simulink model "TCU_Final"  (R2025b)
settings: Solver=FixedStepDiscrete  StartTime=0.0  StopTime=inf  RelTol=1e-3
libraries: TCU_GS x1, TCU_HPC x1
settings Model: Creator=Jairs  LastModifiedBy=joshu
settings OptimizationCC: DefaultParameterBehavior=Inlined  EnhancedBackFolding=on  PassReuseOutputArgsAs=Individual arguments  ZeroExternalMemoryAtStartup=off  ZeroInternalMemoryAtStartup=off  OptimizeBlockOrder=speed  DifferentSizesBufferReuse=on  OptimizationCustomize=off  EfficientTunableParamExpr=on
settings DebuggingCC: ParameterTunabilityLossMsg=error
settings HardwareCC: ProdBitPerPointer=32.0  ProdBitPerSizeT=32.0  ProdBitPerPtrDiffT=32.0  ProdLargestAtomicInteger=Long  ProdLargestAtomicFloat=Double  ProdWordSize=32.0  ProdHWDeviceType=ARM Compatible->ARM Cortex-M
settings SFSimCC: MATLABDynamicMemAlloc=off
settings RTWCC: SystemTargetFile=ert.tlc  GenCodeOnly=on  TemplateMakefile=ert_default_tmf  Description=Embedded Coder
settings CodeAppCC: ForceParamTrailComments=on  IgnoreCustomStorageClasses=off  OperatorAnnotations=on  SimulinkDataObjDesc=on  SFDataObjDesc=on  InsertBlockDesc=on
settings ERTTargetCC: ERTCustomFileTemplate=example_file_process.tlc  TargetLangStandard=C99 (ISO)  GenerateSampleERTMain=on

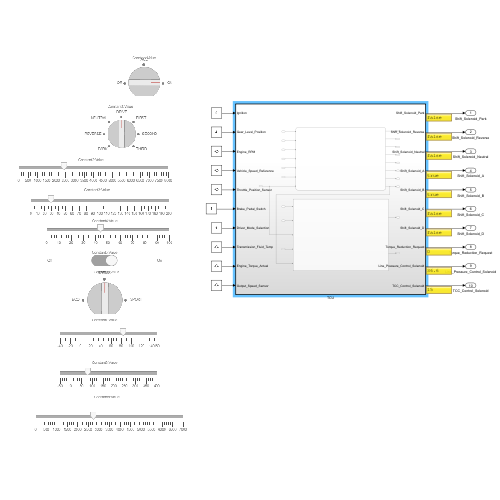
[thumbnail: Simulink's stored preview of the top-level diagram]
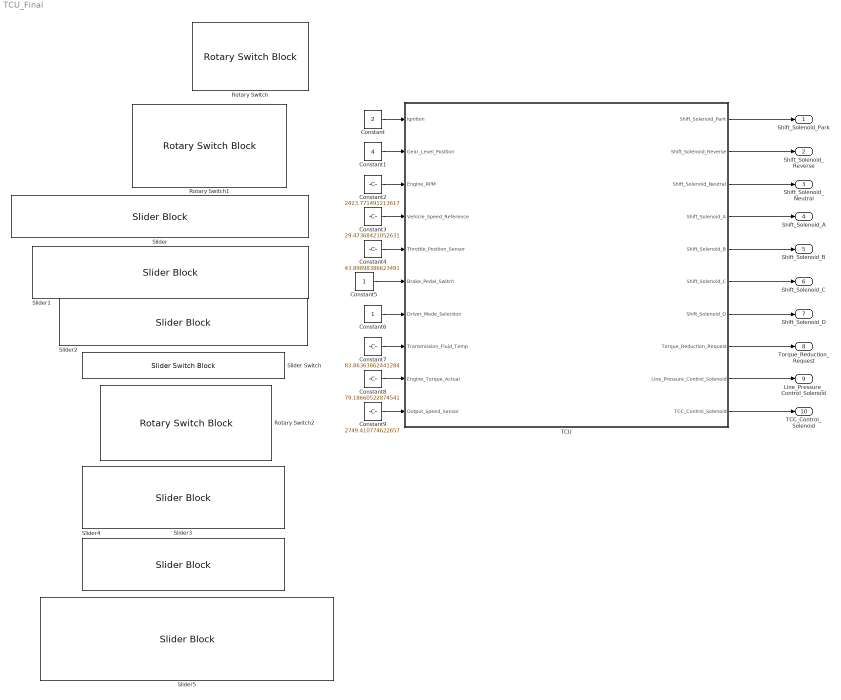
== system TCU_Final ==
  Constant : Constant  Value=2
  Constant1 : Constant  Value=4
  Constant2 : Constant  Value=2423.771491213617
  Constant3 : Constant  Value=29.47368421052631
  Constant4 : Constant  Value=43.89898386623491
  Constant5 : Constant  OutDataTypeStr=boolean
  Constant6 : Constant
  Constant7 : Constant  Value=83.86363862441284
  Constant8 : Constant  Value=79.18660522874541
  Constant9 : Constant  Value=2749.410774622657
  Rotary Switch : RotarySwitchBlock
  Rotary Switch1 : RotarySwitchBlock
  Rotary Switch2 : RotarySwitchBlock
  Slider : SliderBlock  ScaleMax=8000  TickInterval=500
  Slider Switch : SliderSwitchBlock
  Slider1 : SliderBlock  ScaleMax=200  TickInterval=10
  Slider2 : SliderBlock  TickInterval=10
  Slider3 : SliderBlock  ScaleMin=-40  ScaleMax=150  TickInterval=20
  Slider4 : SliderBlock  ScaleMin=-50  ScaleMax=400  TickInterval=50
  Slider5 : SliderBlock  ScaleMax=7000  TickInterval=500
  TCU : Subsystem  TreatAsAtomicUnit=on
      settings: RTWFcnNameOpts=Use subsystem name  RTWFileNameOpts=Use subsystem name
  Shift_Solenoid_Park : Outport
  Shift_Solenoid_Reverse : Outport  Port=2
  Shift_Solenoid_Neutral : Outport  Port=3
  Shift_Solenoid_A : Outport  Port=4
  Shift_Solenoid_B : Outport  Port=5
  Shift_Solenoid_C : Outport  Port=6
  Shift_Solenoid_D : Outport  Port=7
  Torque_Reduction_Request : Outport  Port=8
  Line_Pressure_Control_Solenoid : Outport  Port=9
  TCC_Control_Solenoid : Outport  Port=10
  wires:
  TCU/10(TCC_Control_Solenoid) -> TCC_Control_Solenoid/1
  TCU/9(Line_Pressure_Control_Solenoid) -> Line_Pressure_Control_Solenoid/1
  TCU/8(Torque_Reduction_Request) -> Torque_Reduction_Request/1
  TCU/7(Shift_Solenoid_D) -> Shift_Solenoid_D/1
  TCU/6(Shift_Solenoid_C) -> Shift_Solenoid_C/1
  TCU/5(Shift_Solenoid_B) -> Shift_Solenoid_B/1
  TCU/4(Shift_Solenoid_A) -> Shift_Solenoid_A/1
  TCU/3(Shift_Solenoid_Neutral) -> Shift_Solenoid_Neutral/1
  TCU/2(Shift_Solenoid_Reverse) -> Shift_Solenoid_Reverse/1
  TCU/1(Shift_Solenoid_Park) -> Shift_Solenoid_Park/1
  Constant9/1 -> TCU/10(Output_Speed_Sensor)
  Constant8/1 -> TCU/9(Engine_Torque_Actual)
  Constant7/1 -> TCU/8(Transmission_Fluid_Temp)
  Constant6/1 -> TCU/7(Driver_Mode_Selection)
  Constant5/1 -> TCU/6(Brake_Pedal_Switch)
  Constant4/1 -> TCU/5(Throttle_Position_Sensor)
  Constant3/1 -> TCU/4(Vehicle_Speed_Reference)
  Constant2/1 -> TCU/3(Engine_RPM)
  Constant1/1 -> TCU/2(Gear_Level_Position)
  Constant/1 -> TCU/1(Ignition)

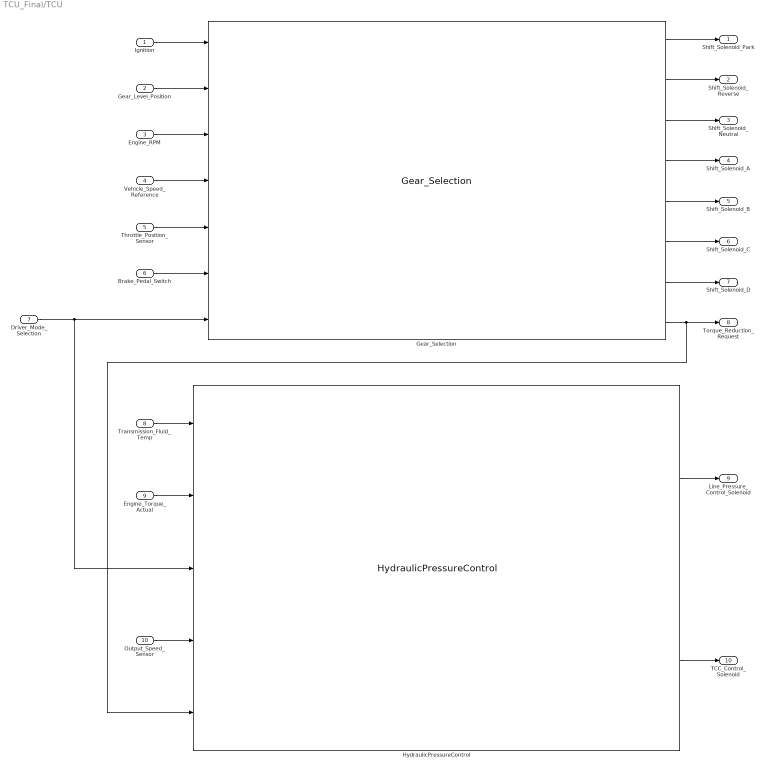
== system TCU_Final/TCU ==
  Ignition : Inport  OutDataTypeStr=double  PortDimensions=1
  Gear_Level_Position : Inport  Port=2  OutDataTypeStr=double  PortDimensions=1
  Engine_RPM : Inport  Port=3  OutDataTypeStr=double  PortDimensions=1
  Vehicle_Speed_Reference : Inport  Port=4  OutDataTypeStr=double  PortDimensions=1
  Throttle_Position_Sensor : Inport  Port=5  OutDataTypeStr=double  PortDimensions=1
  Brake_Pedal_Switch : Inport  Port=6  OutDataTypeStr=boolean  PortDimensions=1
  Driver_Mode_Selection : Inport  Port=7  OutDataTypeStr=double  PortDimensions=1
  Transmission_Fluid_Temp : Inport  Port=8  OutDataTypeStr=double  PortDimensions=1
  Engine_Torque_Actual : Inport  Port=9  OutDataTypeStr=double  PortDimensions=1
  Output_Speed_Sensor : Inport  Port=10  OutDataTypeStr=double  PortDimensions=1
  Gear_Selection : TCU_GS/Gear_Selection  SystemSampleTime=-1  VariantActivationTime=update diagram  EmptyChoice=off  PassThrough=off  PassThroughVariantControl=(default)  EmptyChoiceVariantControl=(default)  AllowFlexibleInterface=on  Latency=0  AutoFrameSizeCalculation=off
  HydraulicPressureControl : TCU_HPC/HydraulicPressureControl  SystemSampleTime=-1  VariantActivationTime=update diagram  EmptyChoice=off  PassThrough=off  PassThroughVariantControl=(default)  EmptyChoiceVariantControl=(default)  AllowFlexibleInterface=on  Latency=0  AutoFrameSizeCalculation=off
  Shift_Solenoid_Park : Outport  OutDataTypeStr=boolean  PortDimensions=1
  Shift_Solenoid_Reverse : Outport  Port=2  OutDataTypeStr=boolean  PortDimensions=1
  Shift_Solenoid_Neutral : Outport  Port=3  OutDataTypeStr=boolean  PortDimensions=1
  Shift_Solenoid_A : Outport  Port=4  OutDataTypeStr=boolean  PortDimensions=1
  Shift_Solenoid_B : Outport  Port=5  OutDataTypeStr=boolean  PortDimensions=1
  Shift_Solenoid_C : Outport  Port=6  OutDataTypeStr=boolean  PortDimensions=1
  Shift_Solenoid_D : Outport  Port=7  OutDataTypeStr=boolean  PortDimensions=1
  Torque_Reduction_Request : Outport  Port=8  OutDataTypeStr=double  PortDimensions=1
  Line_Pressure_Control_Solenoid : Outport  Port=9  OutDataTypeStr=double  PortDimensions=1
  TCC_Control_Solenoid : Outport  Port=10  OutDataTypeStr=double  PortDimensions=1
  wires:
  Ignition/1 -> Gear_Selection/1
  Gear_Level_Position/1 -> Gear_Selection/2
  Engine_RPM/1 -> Gear_Selection/3
  Vehicle_Speed_Reference/1 -> Gear_Selection/4
  Throttle_Position_Sensor/1 -> Gear_Selection/5
  Brake_Pedal_Switch/1 -> Gear_Selection/6
  Driver_Mode_Selection/1 -> Gear_Selection/7, HydraulicPressureControl/3
  Gear_Selection/1 -> Shift_Solenoid_Park/1
  Gear_Selection/3 -> Shift_Solenoid_Neutral/1
  Gear_Selection/2 -> Shift_Solenoid_Reverse/1
  Gear_Selection/4 -> Shift_Solenoid_A/1
  Gear_Selection/5 -> Shift_Solenoid_B/1
  Gear_Selection/6 -> Shift_Solenoid_C/1
  Gear_Selection/7 -> Shift_Solenoid_D/1
  Transmission_Fluid_Temp/1 -> HydraulicPressureControl/1
  Engine_Torque_Actual/1 -> HydraulicPressureControl/2
  Output_Speed_Sensor/1 -> HydraulicPressureControl/4
  Gear_Selection/8 -> HydraulicPressureControl/5, Torque_Reduction_Request/1
  HydraulicPressureControl/1 -> Line_Pressure_Control_Solenoid/1
  HydraulicPressureControl/2 -> TCC_Control_Solenoid/1
